simulink model "syncGenInfBusSimulink"  (R2013a)
settings: Solver=ode45  StartTime=0.0  StopTime=10.0  RelTol=1e-3
undefined symbols (not defined in the file): D_p, gamma, J, L_f, L_s, m, R_f, R_s
settings Model: Creator=USER  LastModifiedBy=USER

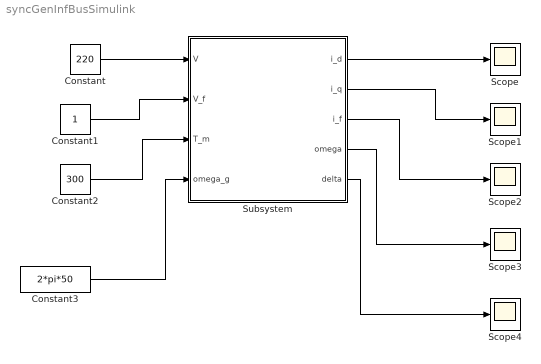
== system syncGenInfBusSimulink ==
  Constant : Constant  Value=220
  Constant1 : Constant
  Constant2 : Constant  Value=300
  Constant3 : Constant  Value=2*pi*50
  Scope{,1..4} (5 alike) : Scope
      Scope2 settings: SaveName=ScopeData2
      Scope3 settings: SaveName=ScopeData3
      Scope4 settings: SaveName=ScopeData4
  Subsystem : Subsystem
  wires:
  Subsystem/1(i_d) -> Scope/1
  Subsystem/2("i_q ") -> Scope1/1
  Subsystem/3(i_f) -> Scope2/1
  Subsystem/4(omega) -> Scope3/1
  Subsystem/5(delta) -> Scope4/1
  Constant/1 -> Subsystem/1(V)
  Constant1/1 -> Subsystem/2(V_f)
  Constant2/1 -> Subsystem/3(T_m)
  Constant3/1 -> Subsystem/4(omega_g)

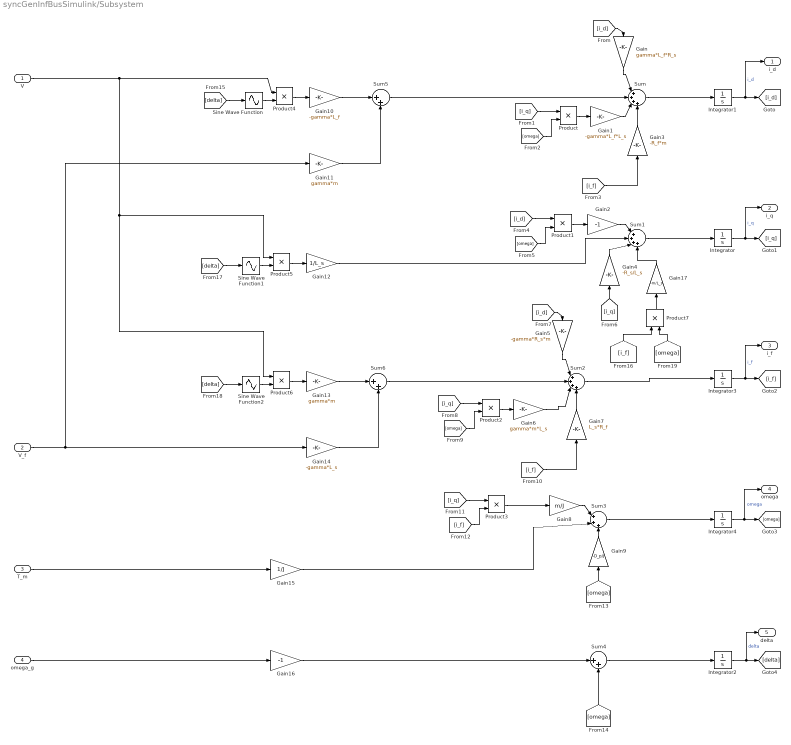
== system syncGenInfBusSimulink/Subsystem ==
  V : Inport
  V_f : Inport  Port=2
  T_m : Inport  Port=3
  omega_g : Inport  Port=4
  Gain : Gain  Gain=gamma*L_f*R_s
  Gain1 : Gain  Gain=-gamma*L_f*L_s
  Gain10 : Gain  Gain=-gamma*L_f
  Gain11 : Gain  Gain=gamma*m
  Gain12 : Gain  Gain=1/L_s
  Gain13 : Gain  Gain=gamma*m
  Gain14 : Gain  Gain=-gamma*L_s
  Gain15 : Gain  Gain=1/J
  Gain16 : Gain  Gain=-1
  Gain17 : Gain  Gain=-m/L_s
  Gain2 : Gain  Gain=-1
  Gain3 : Gain  Gain=-R_f*m
  Gain4 : Gain  Gain=-R_s/L_s
  Gain5 : Gain  Gain=-gamma*R_s*m
  Gain6 : Gain  Gain=gamma*m*L_s
  Gain7 : Gain  Gain=L_s*R_f
  Gain8 : Gain  Gain=m/J
  Gain9 : Gain  Gain=-D_p/J
  Integrator{,1..3} (4 alike) : Integrator
  Integrator4 : Integrator  InitialCondition=2*pi*50
  Product{,1..7} (8 alike) : Product
  Sine Wave Function : Sin  TimeSource=Use external signal  Phase=pi/2  SampleTime=0
  Sine Wave Function1 : Sin  TimeSource=Use external signal  SampleTime=0
  Sine Wave Function2 : Sin  TimeSource=Use external signal  Phase=pi/2  SampleTime=0
  Sum : Sum  Inputs=|++++
  Sum1 : Sum  Inputs=|++++
  Sum2 : Sum  Inputs=|++++
  Sum3 : Sum  Inputs=|+++
  Sum4 : Sum  Inputs=|++
  Sum5 : Sum  Inputs=|++
  Sum6 : Sum  Inputs=|++
  i_d : Outport
  "i_q " : Outport  Port=2
  i_f : Outport  Port=3
  omega : Outport  Port=4
  delta : Outport  Port=5
  wires:
  Integrator1/1 -> i_d/1, [i_d]  "i_d"
  Integrator/1 -> "i_q "/1, [i_q]  "i_q"
  Integrator3/1 -> i_f/1, [i_f]  "i_f"
  Integrator4/1 -> omega/1, [omega]  "omega"
  Integrator2/1 -> delta/1, [delta]  "delta"
  Sum/1 -> Integrator1/1
  [i_d] -> Gain/1
  Gain/1 -> Sum/1
  Product/1 -> Gain1/1
  [i_q] -> Product/1
  [omega] -> Product/2
  Gain1/1 -> Sum/3
  Gain3/1 -> Sum/4
  [i_f] -> Gain3/1
  Sum1/1 -> Integrator/1
  Gain2/1 -> Sum1/1
  Product1/1 -> Gain2/1
  [i_d] -> Product1/1
  [omega] -> Product1/2
  Gain4/1 -> Sum1/3
  [i_q] -> Gain4/1
  Sum2/1 -> Integrator3/1
  [i_d] -> Gain5/1
  Gain5/1 -> Sum2/1
  Product2/1 -> Gain6/1
  [i_q] -> Product2/1
  [omega] -> Product2/2
  Gain6/1 -> Sum2/3
  Gain7/1 -> Sum2/4
  [i_f] -> Gain7/1
  Sum3/1 -> Integrator4/1
  Gain8/1 -> Sum3/1
  Gain9/1 -> Sum3/3
  [omega] -> Gain9/1
  Product3/1 -> Gain8/1
  [i_q] -> Product3/1
  [i_f] -> Product3/2
  Sum4/1 -> Integrator2/1
  [omega] -> Sum4/2
  Sum5/1 -> Sum/2
  Sine Wave Function/1 -> Product4/2
  [delta] -> Sine Wave Function/1
  Product4/1 -> Gain10/1
  Gain10/1 -> Sum5/1
  V_f/1 -> Gain11/1, Gain14/1
  Gain11/1 -> Sum5/2
  Gain12/1 -> Sum1/2
  Sine Wave Function1/1 -> Product5/2
  [delta] -> Sine Wave Function1/1
  Product5/1 -> Gain12/1
  Sum6/1 -> Sum2/2
  Sine Wave Function2/1 -> Product6/2
  [delta] -> Sine Wave Function2/1
  V/1 -> Product6/1, Product5/1, Product4/1
  Product6/1 -> Gain13/1
  Gain13/1 -> Sum6/1
  Gain14/1 -> Sum6/2
  T_m/1 -> Gain15/1
  Gain15/1 -> Sum3/2
  omega_g/1 -> Gain16/1
  Gain16/1 -> Sum4/1
  Product7/1 -> Gain17/1
  [i_f] -> Product7/1
  [omega] -> Product7/2
  Gain17/1 -> Sum1/4
